simulink model "Simulation"  (R2020b)
settings: Solver=FixedStepAuto  StartTime=0.0  StopTime=100  FixedStep=0.01  MaxStep=0.01  RelTol=1e-3  AbsTol=1e-6  EnableMultiTasking=on
model workspace (MAT data in the model file):
  w1 = 20
  w2 = 10
  w3 = 20
  w4 = 10
  w5 = 20
  w6 = 10
libraries: simulink_extras x15, cstblocks x9, robotmaniplib x3
settings Model: ExtModeTrigMode=oneshot  ExtModeArmWhenConnect=off  Creator=fidan  LastModifiedBy=hanna
settings DataIOCC: SaveFormat=Array  ReturnWorkspaceOutputs=off
settings OptimizationCC: BooleanDataType=off
settings DebuggingCC: SaveWithParameterizedLinksMsg=none  UnderspecifiedInitializationDetection=Classic  MergeDetectMultiDrivingBlocksExec=none  SignalResolutionControl=TryResolveAllWithWarning  MultiTaskDSMMsg=warning  MultiTaskCondExecSysMsg=none  ArithmeticOperatorsInVariantConditions=warning
settings HardwareCC: TargetBitPerPointer=64  TargetBitPerSizeT=64  TargetBitPerPtrDiffT=64  TargetLongLongMode=on  TargetIntDivRoundTo=Zero  TargetEndianess=LittleEndian  TargetWordSize=64  TargetHWDeviceType=MATLAB Host  ProdEqTarget=off
settings ModelReferenceCC: PropagateSignalLabelsOutOfModel=off
settings SFSimCC: CustomCodeUndefinedFunction=UseInterfaceOnly
settings RTWCC: GenCodeOnly=on
settings GRTTargetCC: CombineOutputUpdateFcns=off  GRTInterface=on
settings ConfigComp: CovMetricSettings=dw

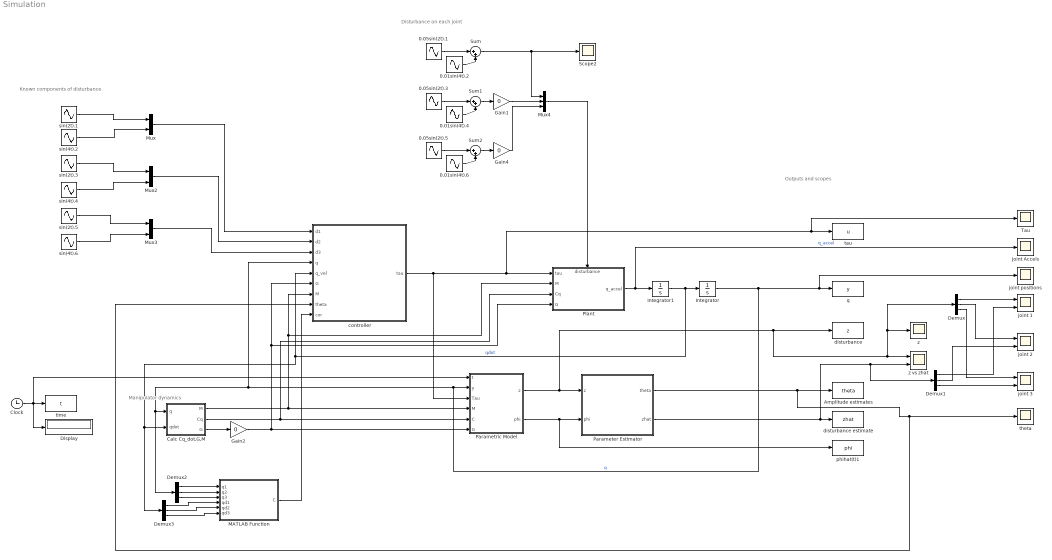
== system Simulation ==
  note: Manipulator dynamics
  note: Known components of disturbance
  note: Outputs and scopes
  note: Disturbance on each joint
  0.01sin(4t).2 : Sin  Amplitude=0.01  Frequency=w2  SampleTime=0
  0.01sin(4t).4 : Sin  Amplitude=0.01  Frequency=w4  SampleTime=0
  0.01sin(4t).6 : Sin  Amplitude=0.01  Frequency=w6  SampleTime=0
  0.05sin(2t).1 : Sin  Amplitude=0.05  Frequency=w1  SampleTime=0
  0.05sin(2t).3 : Sin  Amplitude=0.05  Frequency=w3  SampleTime=0
  0.05sin(2t).5 : Sin  Amplitude=0.05  Frequency=w5  SampleTime=0
  Amplitude estimates : ToWorkspace  VariableName=theta  SampleTime=-1
  Calc Cq_dot,G,M : Subsystem
  Clock : Clock
  Demux{,1..3} (4 alike) : Demux  Outputs=3
  Display : Display
  Gain1 : Gain  Gain=0
  Gain2 : Gain  Gain=0
  Gain4 : Gain  Gain=0
  Integrator : Integrator  InitialCondition=[0.1 0.1 0.1]
  Integrator1 : Integrator  InitialCondition=[0 0 0]
  Joint Accels : Scope
  MATLAB Function : MATLAB Function  TreatAsAtomicUnit=on
  Mux : Mux  Inputs=2
  Mux2 : Mux  Inputs=2
  Mux3 : Mux  Inputs=2
  Mux4 : Mux  Inputs=3
  Parameter Estimator : Subsystem  TreatAsAtomicUnit=on
  Parametric Model : Subsystem  TreatAsAtomicUnit=on
  Plant : Subsystem  TreatAsAtomicUnit=on
      settings: PortSchema="{\"entries\":[{\"content\":{\"sides\":[{\"content\":{\"connectorIds\":[\"In1\",\"In2\",\"In3\",\"In4\"]},\"type\":\"ConnectorPlacement.EquallySpacedRectSide\",\"uuid\":\"686171d9-bf50-46f5-8d0d-4031646190b8\"},{\"content\":{\"connectorIds\":[\"Out1\"],\"side\":\"RIGHT\"},\"type\":\"ConnectorPlacement.EquallySpacedRectSide\",\"uuid\":\"2d2db6b0-29ef-468f-b4f6-9a6a72123182\"},{\"content\":{\"connectorIds\":[\"In5\"],\"side\":\"TOP\"},\"type\":\"ConnectorPlacement.EquallySpacedRectSide\",\"uuid\":\"df4eb408-a400-4123-8352-c11ce71c265d\"}]},\"type\":\"ConnectorPlacement.EquallySpacedConnector\",\"uuid\":\"e3a00764-9db2-4b17-91fa-1626c36d3d40\"}],\"packageUris\":[\"http://schema.mathworks.com/mf0/Connector/19700101\"],\"version\":\"1.0\"}"
  Scope2 : Scope
  Sum : Sum  Inputs=|++
  Sum1 : Sum  Inputs=|++
  Sum2 : Sum  Inputs=|++
  Tau : Scope
  controller : MATLAB Function  TreatAsAtomicUnit=on
  disturbance : ToWorkspace  VariableName=z  SampleTime=-1
  disturbance estimate : ToWorkspace  VariableName=zhat  SampleTime=-1
  joint 1 : Scope  NumInputPorts=2
  joint 2 : Scope  NumInputPorts=2
  joint 3 : Scope  NumInputPorts=2
  joint positions : Scope
  phihat(t)1 : ToWorkspace  VariableName=phi  SampleTime=-1
  q : ToWorkspace  VariableName=y  SampleTime=-1
  sin(2t).1 : Sin  Frequency=w1  SampleTime=0
  sin(2t).3 : Sin  Frequency=w3  SampleTime=0
  sin(2t).5 : Sin  Frequency=w5  SampleTime=0
  sin(4t).2 : Sin  Frequency=w2  SampleTime=0
  sin(4t).4 : Sin  Frequency=w4  SampleTime=0
  sin(4t).6 : Sin  Frequency=w6  SampleTime=0
  tau : ToWorkspace  VariableName=u  SampleTime=-1
  theta : Scope
  time : ToWorkspace  VariableName=t  SampleTime=-1
  z : Scope
  z vs zhat : Scope  NumInputPorts=2
  wires:
  Mux4/1 -> Plant/5(disturbance)
  Parametric Model/2(phi) -> phihat(t)1/1, Parameter Estimator/2(phi)
  Parameter Estimator/1(theta) -> controller/8(theta), theta/1, Amplitude estimates/1
  controller/1(tau) -> Parametric Model/3(Tau), tau/1, Tau/1, Plant/1(tau)
  0.05sin(2t).1/1 -> Sum/1
  0.01sin(4t).2/1 -> Sum/2
  0.01sin(4t).4/1 -> Sum1/2
  0.05sin(2t).3/1 -> Sum1/1
  0.05sin(2t).5/1 -> Sum2/1
  0.01sin(4t).6/1 -> Sum2/2
  Sum2/1 -> Gain4/1
  Integrator1/1 -> Demux3/1, Calc Cq_dot,G,M/2(qdot), controller/5(q_vel), Integrator/1  "qdot"
  Integrator/1 -> joint positions/1, q/1, Parametric Model/2(y), Demux2/1, Calc Cq_dot,G,M/1(q), controller/4(q)  "q"
  Calc Cq_dot,G,M/1(M) -> controller/7(M), Plant/2(M), Parametric Model/4(M)
  Plant/1(q_accel) -> Joint Accels/1, Integrator1/1  "q_accel"
  Demux/1 -> joint 1/1
  Calc Cq_dot,G,M/3(G) -> Gain2/1
  Demux1/1 -> joint 1/2
  Demux/2 -> joint 2/1
  Demux1/2 -> joint 2/2
  Demux/3 -> joint 3/1
  Demux1/3 -> joint 3/2
  MATLAB Function/1(C) -> controller/9(cor)
  Demux2/1 -> MATLAB Function/1(q1)
  Demux2/2 -> MATLAB Function/2(q2)
  Demux2/3 -> MATLAB Function/3(q3)
  Demux3/1 -> MATLAB Function/4(qd1)
  Demux3/2 -> MATLAB Function/5(qd2)
  Demux3/3 -> MATLAB Function/6(qd3)
  Clock/1 -> Display/1, Parametric Model/1(t), time/1
  Sum1/1 -> Gain1/1
  Sum/1 -> Mux4/1, Scope2/1
  Parameter Estimator/2(zhat) -> Demux1/1, z vs zhat/2, disturbance estimate/1
  Gain1/1 -> Mux4/2
  Gain4/1 -> Mux4/3
  Gain2/1 -> Plant/4(G), controller/6(G), Parametric Model/6(G)
  Calc Cq_dot,G,M/2(Cq) -> Plant/3(Cq), Parametric Model/5(C)
  Parametric Model/1(z) -> z vs zhat/1, Demux/1, z/1, disturbance/1, Parameter Estimator/1(z)
  sin(2t).1/1 -> Mux/1
  sin(4t).2/1 -> Mux/2
  sin(2t).3/1 -> Mux2/1
  sin(4t).4/1 -> Mux2/2
  sin(2t).5/1 -> Mux3/1
  sin(4t).6/1 -> Mux3/2
  Mux/1 -> controller/1(d1)
  Mux2/1 -> controller/2(d2)
  Mux3/1 -> controller/3(d3)

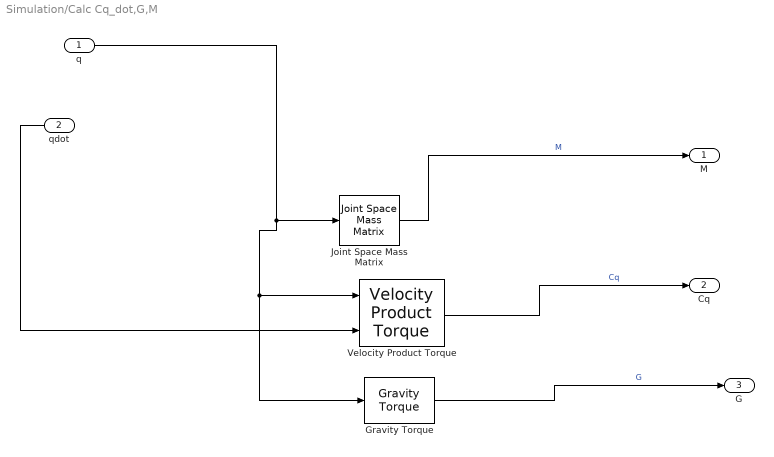
== system Simulation/Calc Cq_dot,G,M ==
  q : Inport
  qdot : Inport  Port=2
  Gravity Torque : robotmaniplib/Gravity Torque  RigidBodyTree=myrobot  SimulateUsing=Interpreted execution
  Joint Space Mass Matrix : robotmaniplib/Joint Space Mass Matrix  RigidBodyTree=myrobot  SimulateUsing=Interpreted execution
  Velocity Product Torque : robotmaniplib/Velocity Product Torque  RigidBodyTree=myrobot  SimulateUsing=Interpreted execution
      settings: SourceProductBaseCode=RO
  M : Outport
  Cq : Outport  Port=2
  G : Outport  Port=3
  wires:
  Velocity Product Torque/1 -> Cq/1  "Cq"
  Joint Space Mass Matrix/1 -> M/1  "M"
  qdot/1 -> Velocity Product Torque/2
  Gravity Torque/1 -> G/1  "G"
  q/1 -> Gravity Torque/1, Velocity Product Torque/1, Joint Space Mass Matrix/1

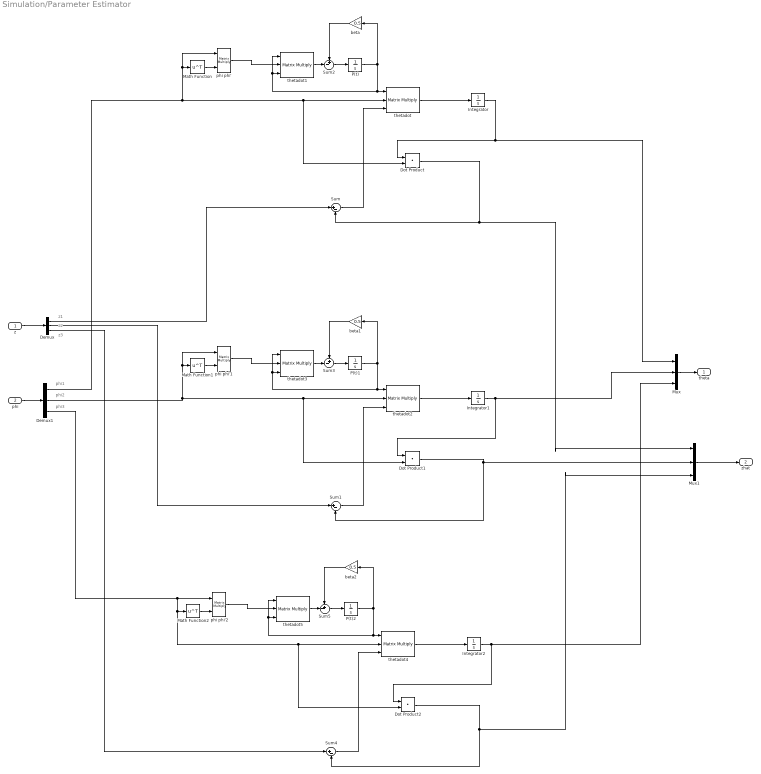
== system Simulation/Parameter Estimator ==
  note: phi3
  note: phi2
  note: phi1
  note: z2
  note: z1
  note: z3
  z : Inport
  phi : Inport  Port=2
  Demux : Demux  Outputs=3
  Demux1 : Demux  Outputs=3
  Dot Product : DotProduct  InputSameDT=on  OutDataTypeStr=Inherit: Inherit via internal rule
  Dot Product1 : DotProduct  InputSameDT=on  OutDataTypeStr=Inherit: Inherit via internal rule
  Dot Product2 : DotProduct  InputSameDT=on  OutDataTypeStr=Inherit: Inherit via internal rule
  Integrator : Integrator  InitialCondition=[0.001 0.001]'
  Integrator1 : Integrator  InitialCondition=[0.001 0.001]'
  Integrator2 : Integrator  InitialCondition=[0.001 0.001]'
  Math Function : Math  Operator=transpose  SignedPower=on  SaturateOnIntegerOverflow=on
  Math Function1 : Math  Operator=transpose  SignedPower=on  SaturateOnIntegerOverflow=on
  Math Function2 : Math  Operator=transpose  SignedPower=on  SaturateOnIntegerOverflow=on
  Mux : Mux  Inputs=3
  Mux1 : Mux  Inputs=3
  P(t) : Integrator  InitialCondition=1*eye(2)
  P(t)1 : Integrator  InitialCondition=1*eye(2)
  P(t)2 : Integrator  InitialCondition=1*eye(2)
  Sum : Sum  Tag=epsilon  Description=epsilon  Inputs=|+-
  Sum1 : Sum  Tag=epsilon  Description=epsilon  Inputs=|+-
  Sum2 : Sum  Tag=epsilon  Description=epsilon  Inputs=+-|
  Sum3 : Sum  Tag=epsilon  Description=epsilon  Inputs=+-|
  Sum4 : Sum  Tag=epsilon  Description=epsilon  Inputs=|+-
  Sum5 : Sum  Tag=epsilon  Description=epsilon  Inputs=+-|
  beta : Gain  Gain=0.5
  beta1 : Gain  Gain=0.5
  beta2 : Gain  Gain=0.5
  phi phi' : Product  Multiplication=Matrix(*)
  phi phi'1 : Product  Multiplication=Matrix(*)
  phi phi'2 : Product  Multiplication=Matrix(*)
  thetadot{,1..5} (6 alike) : Product  Inputs=3  Multiplication=Matrix(*)
  theta : Outport  VectorParamsAs1DForOutWhenUnconnected=off
  zhat : Outport  Port=2  VectorParamsAs1DForOutWhenUnconnected=off
  wires:
  z/1 -> Demux/1
  phi phi'/1 -> thetadot1/2
  P(t)/1 -> thetadot/1, thetadot1/3, thetadot1/1, beta/1
  Sum2/1 -> P(t)/1
  thetadot1/1 -> Sum2/2
  thetadot/1 -> Integrator/1
  beta/1 -> Sum2/1
  Math Function/1 -> phi phi'/2
  Demux1/1 -> phi phi'/1, Math Function/1, Dot Product/2, thetadot/2
  Integrator/1 -> Mux/1, Dot Product/1
  Demux/1 -> Sum/1
  Sum/1 -> thetadot/3
  Demux/2 -> Sum1/1
  Demux1/2 -> phi phi'1/1, Math Function1/1, Dot Product1/2, thetadot2/2
  Sum1/1 -> thetadot2/3
  P(t)1/1 -> thetadot2/1, thetadot3/3, thetadot3/1, beta1/1
  Sum3/1 -> P(t)1/1
  Integrator1/1 -> Mux/2, Dot Product1/1
  thetadot2/1 -> Integrator1/1
  beta1/1 -> Sum3/1
  Math Function1/1 -> phi phi'1/2
  thetadot3/1 -> Sum3/2
  phi phi'1/1 -> thetadot3/2
  Sum4/1 -> thetadot4/3
  Integrator2/1 -> Mux/3, Dot Product2/1
  P(t)2/1 -> thetadot4/1, thetadot5/3, thetadot5/1, beta2/1
  Sum5/1 -> P(t)2/1
  Demux1/3 -> Dot Product2/2, thetadot4/2, Math Function2/1, phi phi'2/1
  phi phi'2/1 -> thetadot5/2
  Math Function2/1 -> phi phi'2/2
  thetadot5/1 -> Sum5/2
  Demux/3 -> Sum4/1
  thetadot4/1 -> Integrator2/1
  beta2/1 -> Sum5/1
  phi/1 -> Demux1/1
  Mux/1 -> theta/1
  Mux1/1 -> zhat/1
  Dot Product1/1 -> Sum1/2, Mux1/2
  Dot Product/1 -> Mux1/1, Sum/2
  Dot Product2/1 -> Mux1/3, Sum4/2

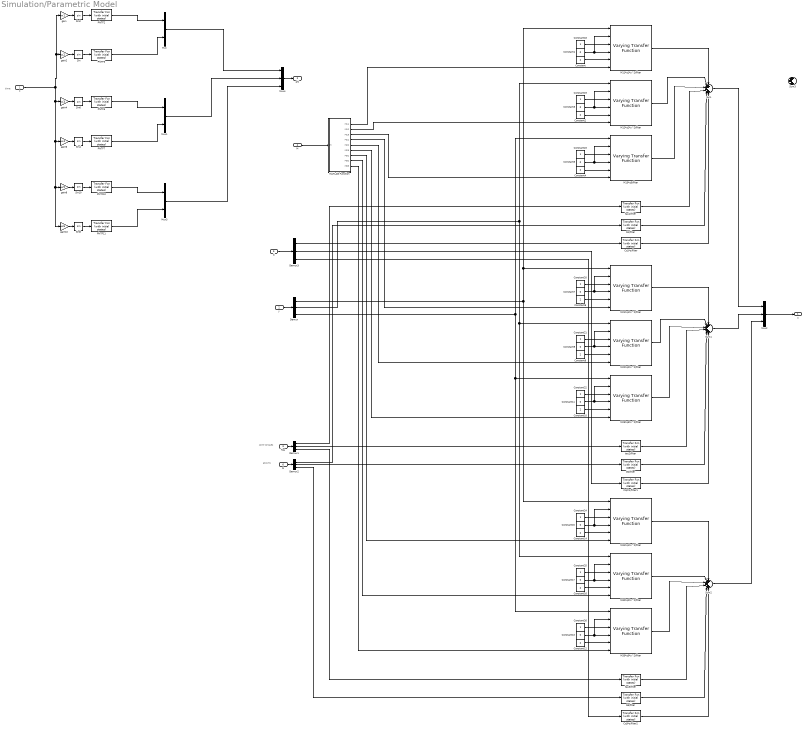
== system Simulation/Parametric Model ==
  note: time
  note: gravity
  note: joint torques
  t : Inport
  y : Inport  Port=2
  Tau : Inport  Port=3
  M : Inport  Port=4
  C : Inport  Port=5
  G : Inport  Port=6
  Constant{,2,4,6,8,10,12,14,16} (9 alike) : Constant  Value=2
  Constant{1,3,5,7,9,11,13,15,17} (9 alike) : Constant  Value=0
  Constant{18..26} (9 alike) : Constant
  Cq1*s/filter : simulink_extras/Additional Linear/Transfer Fcn (with initial states)  N=[1 0]  D=[1 2 1]  X0=0
  Cq2*s/filter1 : simulink_extras/Additional Linear/Transfer Fcn (with initial states)  N=[1 0]  D=[1 2 1]  X0=0
  Cq3*s/filter2 : simulink_extras/Additional Linear/Transfer Fcn (with initial states)  N=[1 0]  D=[1 2 1]  X0=0
  Demux{,1..3} (4 alike) : Demux  Outputs=3
  G1/filter : simulink_extras/Additional Linear/Transfer Fcn (with initial states)  N=[1]  D=[1 2 1]  X0=0
  G2/filter : simulink_extras/Additional Linear/Transfer Fcn (with initial states)  N=[1]  D=[1 2 1]  X0=0
  G3/filter : simulink_extras/Additional Linear/Transfer Fcn (with initial states)  N=[1]  D=[1 2 1]  X0=0
  M11*q1*s^2/filter : cstblocks/Linear Parameter Varying/Varying Transfer Function  N=2
  M12*q2*s^2/filter : cstblocks/Linear Parameter Varying/Varying Transfer Function  N=2
  M13*q3/filter : cstblocks/Linear Parameter Varying/Varying Transfer Function  N=2
  M21*q1*s^2/filter : cstblocks/Linear Parameter Varying/Varying Transfer Function  N=2
  M22*q2*s^2/filter : cstblocks/Linear Parameter Varying/Varying Transfer Function  N=2
  M23*q3*s^2/filter : cstblocks/Linear Parameter Varying/Varying Transfer Function  N=2
  M31*q1*s^2/filter : cstblocks/Linear Parameter Varying/Varying Transfer Function  N=2
  M32*q2*s^2/filter : cstblocks/Linear Parameter Varying/Varying Transfer Function  N=2
  M33*q3*s^2/filter : cstblocks/Linear Parameter Varying/Varying Transfer Function  N=2
  MATLAB Function : MATLAB Function  TreatAsAtomicUnit=on
  Mux : Mux  Inputs=2
  Mux1 : Mux  Inputs=2
  Mux2 : Mux  Inputs=3
  Mux3 : Mux  Inputs=2
  Mux4 : Mux  Inputs=3
  PhiTF{2..3,5,7,10..11} (6 alike) : simulink_extras/Additional Linear/Transfer Fcn (with initial states)  N=[1]  D=[1 2 1]  X0=0
  Sin{,2,4,6,8,10} (6 alike) : Trigonometry
  Sum{,1..3} (4 alike) : Sum  Inputs=+++-++
  gain : Gain  Gain=w1
  gain10 : Gain  Gain=w6
  gain2 : Gain  Gain=w2
  gain4 : Gain  Gain=w3
  gain6 : Gain  Gain=w4
  gain8 : Gain  Gain=w5
  tau1/filter : simulink_extras/Additional Linear/Transfer Fcn (with initial states)  N=[1]  D=[1 2 1]  X0=0
  tau2/filter : simulink_extras/Additional Linear/Transfer Fcn (with initial states)  N=[1]  D=[1 2 1]  X0=0
  tau3/filter : simulink_extras/Additional Linear/Transfer Fcn (with initial states)  N=[1]  D=[1 2 1]  X0=0
  z : Outport  VectorParamsAs1DForOutWhenUnconnected=off
  phi : Outport  Port=2  VectorParamsAs1DForOutWhenUnconnected=off
  wires:
  PhiTF2/1 -> Mux/1
  y/1 -> Demux/1
  Cq1*s/filter/1 -> Sum/6
  Mux/1 -> Mux4/1
  PhiTF3/1 -> Mux/2
  Sin/1 -> PhiTF3/1
  gain2/1 -> Sin/1
  gain/1 -> Sin2/1
  Sin2/1 -> PhiTF2/1
  t/1 -> gain2/1, gain/1, gain10/1, gain8/1, gain6/1, gain4/1
  gain4/1 -> Sin6/1
  Sin4/1 -> PhiTF7/1
  Sin6/1 -> PhiTF5/1
  gain6/1 -> Sin4/1
  PhiTF7/1 -> Mux1/2
  PhiTF5/1 -> Mux1/1
  gain8/1 -> Sin10/1
  Sin8/1 -> PhiTF11/1
  Sin10/1 -> PhiTF10/1
  gain10/1 -> Sin8/1
  PhiTF11/1 -> Mux3/2
  PhiTF10/1 -> Mux3/1
  Mux1/1 -> Mux4/2
  Mux3/1 -> Mux4/3
  M12*q2*s^2/filter/1 -> Sum/2
  M13*q3/filter/1 -> Sum/3
  Sum/1 -> Mux2/1
  Tau/1 -> Demux1/1
  Demux1/1 -> tau1/filter/1
  tau1/filter/1 -> Sum/4
  G/1 -> Demux2/1
  Demux2/1 -> G1/filter/1
  G1/filter/1 -> Sum/5
  C/1 -> Demux3/1
  M/1 -> MATLAB Function/1(M)
  MATLAB Function/1(M11) -> M11*q1*s^2/filter/6
  Demux3/1 -> Cq1*s/filter/1
  Constant/1 -> M11*q1*s^2/filter/5
  Constant1/1 -> M11*q1*s^2/filter/2, M11*q1*s^2/filter/4
  Constant2/1 -> M12*q2*s^2/filter/5
  Constant3/1 -> M12*q2*s^2/filter/2, M12*q2*s^2/filter/4
  Constant4/1 -> M13*q3/filter/5
  Constant5/1 -> M13*q3/filter/2, M13*q3/filter/4
  Constant9/1 -> M22*q2*s^2/filter/4, M22*q2*s^2/filter/2
  Constant8/1 -> M22*q2*s^2/filter/5
  Constant10/1 -> M23*q3*s^2/filter/5
  tau2/filter/1 -> Sum1/4
  Constant11/1 -> M23*q3*s^2/filter/2, M23*q3*s^2/filter/4
  Constant6/1 -> M21*q1*s^2/filter/5
  M21*q1*s^2/filter/1 -> Sum1/1
  M22*q2*s^2/filter/1 -> Sum1/2
  M23*q3*s^2/filter/1 -> Sum1/3
  G2/filter/1 -> Sum1/5
  Constant7/1 -> M21*q1*s^2/filter/2, M21*q1*s^2/filter/4
  MATLAB Function/2(M12) -> M12*q2*s^2/filter/6
  MATLAB Function/3(M13) -> M13*q3/filter/6
  MATLAB Function/4(M21) -> M21*q1*s^2/filter/6
  MATLAB Function/5(M22) -> M22*q2*s^2/filter/6
  MATLAB Function/6(M23) -> M23*q3*s^2/filter/6
  Demux1/2 -> tau2/filter/1
  Demux2/2 -> G2/filter/1
  Sum1/1 -> Mux2/2
  G3/filter/1 -> Sum2/5
  M33*q3*s^2/filter/1 -> Sum2/3
  M32*q2*s^2/filter/1 -> Sum2/2
  M31*q1*s^2/filter/1 -> Sum2/1
  Constant17/1 -> M32*q2*s^2/filter/2, M32*q2*s^2/filter/4
  Constant14/1 -> M31*q1*s^2/filter/5
  Constant13/1 -> M33*q3*s^2/filter/2, M33*q3*s^2/filter/4
  tau3/filter/1 -> Sum2/4
  Constant16/1 -> M32*q2*s^2/filter/5
  Constant15/1 -> M31*q1*s^2/filter/2, M31*q1*s^2/filter/4
  Constant12/1 -> M33*q3*s^2/filter/5
  Demux/1 -> M11*q1*s^2/filter/1, M21*q1*s^2/filter/1, M31*q1*s^2/filter/1
  Demux/2 -> M32*q2*s^2/filter/1, M22*q2*s^2/filter/1, M12*q2*s^2/filter/1
  Demux/3 -> M13*q3/filter/1, M33*q3*s^2/filter/1, M23*q3*s^2/filter/1
  MATLAB Function/7(M31) -> M31*q1*s^2/filter/6
  MATLAB Function/8(M32) -> M32*q2*s^2/filter/6
  MATLAB Function/9(M33) -> M33*q3*s^2/filter/6
  Demux1/3 -> tau3/filter/1
  Demux2/3 -> G3/filter/1
  Sum2/1 -> Mux2/3
  Mux4/1 -> phi/1
  Constant18/1 -> M11*q1*s^2/filter/3
  M11*q1*s^2/filter/1 -> Sum/1
  Constant19/1 -> M12*q2*s^2/filter/3
  Constant20/1 -> M21*q1*s^2/filter/3
  Constant21/1 -> M22*q2*s^2/filter/3
  Constant22/1 -> M23*q3*s^2/filter/3
  Cq2*s/filter1/1 -> Sum1/6
  Constant23/1 -> M13*q3/filter/3
  Demux3/2 -> Cq2*s/filter1/1
  Constant24/1 -> M31*q1*s^2/filter/3
  Constant25/1 -> M32*q2*s^2/filter/3
  Constant26/1 -> M33*q3*s^2/filter/3
  Cq3*s/filter2/1 -> Sum2/6
  Demux3/3 -> Cq3*s/filter2/1
  Mux2/1 -> z/1

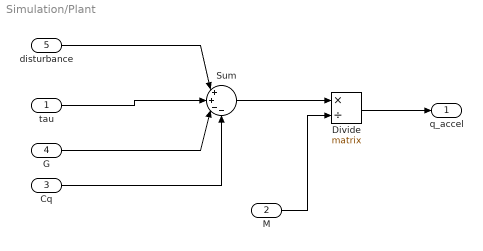
== system Simulation/Plant ==
  tau : Inport
  M : Inport  Port=2
  Cq : Inport  Port=3
  G : Inport  Port=4
  disturbance : Inport  Port=5
  Divide : Product  Inputs=*/  Multiplication=Matrix(*)
  Sum : Sum  Inputs=|++--
  q_accel : Outport  VectorParamsAs1DForOutWhenUnconnected=off
  wires:
  Cq/1 -> Sum/4
  disturbance/1 -> Sum/1
  tau/1 -> Sum/2
  G/1 -> Sum/3
  M/1 -> Divide/2
  Sum/1 -> Divide/1
  Divide/1 -> q_accel/1

== matlab function Simulation/controller ==
  data: d1 input; d2 input; d3 input; q input; q_vel input; G input; M input; tau output; theta input; cor input
function tau = fcn(d1,d2,d3, q, q_vel,G, M, theta, cor)
% POLE PLACEMENT

coder.extrinsic('place')

A = [ zeros(3,3), eye(3);
      eye(3),    -inv(M)*cor ];

B = [ zeros(3,3);
      inv(M) ];

C = [ones(1,3), zeros(1,3)];


%calculate controller gain
Kc11 = 0;
Kc12 = 0;
Kc13 = 0;
Kc14 = 0;
Kc15 = 0;
Kc16 = 0;
Kc21 = 0;
Kc22 = 0;
Kc23 = 0;
Kc24 = 0;
Kc25 = 0;
Kc26 = 0;
Kc31 = 0;
Kc32 = 0;
Kc33 = 0;
Kc34 = 0;
Kc35 = 0;
Kc36 = 0;
% Kc = place(A,B,[-1,-2,-3,-4,-5,-6]');
% Kc = place(A,B,[-6,-6,-5,-5,-2,-2]');
p = [-6,-6,-5,-5,-2,-2]';
Kc = place(A,B,p);

Kc11 = Kc(1,1);
Kc12 = Kc(1,2);
Kc13 = Kc(1,3);
Kc14 = Kc(1,4);
Kc15 = Kc(1,5);
Kc16 = Kc(1,6);
Kc21 = Kc(2,1);
Kc22 = Kc(2,2);
Kc23 = Kc(2,3);
Kc24 = Kc(2,4);
Kc25 = Kc(2,5);
Kc26 = Kc(2,6);
Kc31 = Kc(3,1);
Kc32 = Kc(3,2);
Kc33 = Kc(3,3);
Kc34 = Kc(3,4);
Kc35 = Kc(3,5);
Kc36 = Kc(3,6);

K = [Kc11 Kc12 Kc13 Kc14 Kc15 Kc16;
     Kc21 Kc22 Kc23 Kc24 Kc25 Kc26;
     Kc31 Kc32 Kc33 Kc34 Kc35 Kc36];

x = [q;q_vel];


theta1 = [theta(1),theta(2)];
theta2 = [theta(3),theta(4)];
theta3 = [theta(5),theta(6)];

F_hat = [theta1*d1; theta2*d2; theta3*d3];

% pole placement with disturbance rejection
tau = -K*x+G+M*q-F_hat;


% tau=0*-F_hat;



end

== matlab function Simulation/Parametric Model/MATLAB Function ==
  data: M input; M11 output; M12 output; M13 output; M21 output; M22 output; M23 output; M31 output; M32 output; M33 output
function [M11,M12,M13,M21,M22,M23,M31,M32,M33] = fcn(M)

M11 = M(1,1);
M12 = M(1,2);
M13 = M(1,3);
M21 = M(2,1);
M22 = M(2,2);
M23 = M(2,3);
M31 = M(3,1);
M32 = M(3,2);
M33 = M(3,3);

== matlab function Simulation/MATLAB Function ==
  data: q1 input; C output; q2 input; q3 input; qd1 input; qd2 input; qd3 input
function C = compute_C_2(q1, q2, q3, qd1, qd2, qd3)
%cor1 = load('coriolis_row_1')
%cor2 = load('coriolis_row_2')
%cor3 = load('coriolis_row_3')
c11 = (7569*qd3*cos(q3)*sin(q3))/320000 - (87*qd3*sin(q3))/1600 - (7569*qd2*sin(2*q2)*cos(q3)^2)/320000 - (569*qd2*sin(2*q2))/3200 - (87*qd2*sin(2*q2)*cos(q3))/800 - (87*qd3*cos(2*q2)*sin(q3))/1600 - (7569*qd3*cos(2*q2)*cos(q3)*sin(q3))/320000;
c12 = (87*qd2*cos(q2)*sin(q3))/800 - (167569*qd3*sin(q2))/320000 - (7569*qd1*cos(2*q3)*sin(2*q2))/640000 - (121369*qd1*sin(2*q2))/640000 - (87*qd1*sin(2*q2)*cos(q3))/800 + (7569*qd2*sin(2*q3)*cos(q2))/320000 + (7569*qd3*cos(2*q3)*sin(q2))/320000;
c13 = (7569*qd2*cos(q3)^2*sin(q2))/160000 - (87*qd3*cos(q2)*sin(q3))/800 - (87*qd1*cos(q2)^2*sin(q3))/800 - (87569*qd2*sin(q2))/160000 + (7569*qd1*cos(q3)*sin(q2)^2*sin(q3))/160000;
c21 = (sin(q2)*(80000*qd3 + 7569*qd3*cos(q3)^2 + 56900*qd1*cos(q2) + 17400*qd3*cos(q3) + 34800*qd1*cos(q2)*cos(q3) + 7569*qd1*cos(q2)*cos(q3)^2))/160000;
c22 = -(87*qd3*sin(q3)*(87*cos(q3) + 200))/160000;
c23 = (qd1*sin(q2))/2 - (87*qd2*sin(q3))/800 + (87*qd1*cos(q3)*sin(q2))/800 - (7569*qd2*cos(q3)*sin(q3))/160000 + (7569*qd1*cos(q3)^2*sin(q2))/160000;
c31 = (87*qd1*cos(q2)^2*sin(q3))/800 - (7569*qd1*cos(q3)*sin(q3))/160000 - (87*qd2*cos(q3)*sin(q2))/800 - (qd2*sin(q2))/2 - (7569*qd2*cos(q3)^2*sin(q2))/160000 + (7569*qd1*cos(q2)^2*cos(q3)*sin(q3))/160000;
c32 = (87*qd2*sin(q3))/800 - (qd1*sin(q2))/2 - (87*qd1*cos(q3)*sin(q2))/800 + (7569*qd2*cos(q3)*sin(q3))/160000 - (7569*qd1*cos(q3)^2*sin(q2))/160000;
c33 = 0;

C = [c11 c12 c13;
     c21 c22 c23;
     c31 c32 c33];
